simulink model "Planner_Operational_Space"  (Simulink 9.3)
settings: Solver=FixedStepDiscrete  StartTime=0.0  StopTime=stop_time  FixedStep=dt  RelTol=1e-3  EnableMultiTasking=on
values from neighbouring files (symbols this model uses):
  Cost = [0.25 0.2 0.25 0.3 start_time1 stop_time1 ]    [initialization.m]
  Cost1 = [0.25 0.3 0.25 0.25 start_time2 stop_time2 ]    [initialization.m]
  Cost2 = [0.25 0.25 0.25 0.2 start_time3 stop_time3 ]    [initialization.m]
  stop_time1 = 4    [initialization.m]
  stop_time2 = 8    [initialization.m]
undefined symbols (not defined in the file or in its folder): circonferenza1, circonferenza2, percorso
libraries: simulink x1
settings Model: Creator=Nino  LastModifiedBy=Simone
settings DataIOCC: LimitDataPoints=on
settings OptimizationCC: ExpressionDepthLimit=2147483647  InitFltsAndDblsToZero=on
settings DebuggingCC: SolverPrmCheckMsg=warning  StateNameClashWarn=warning  PregeneratedLibrarySubsystemCodeDiagnostic=none
settings GRTTargetCC: GeneratePreprocessorConditionals=Disable all
settings ConfigComp: CovSFcnEnable=off

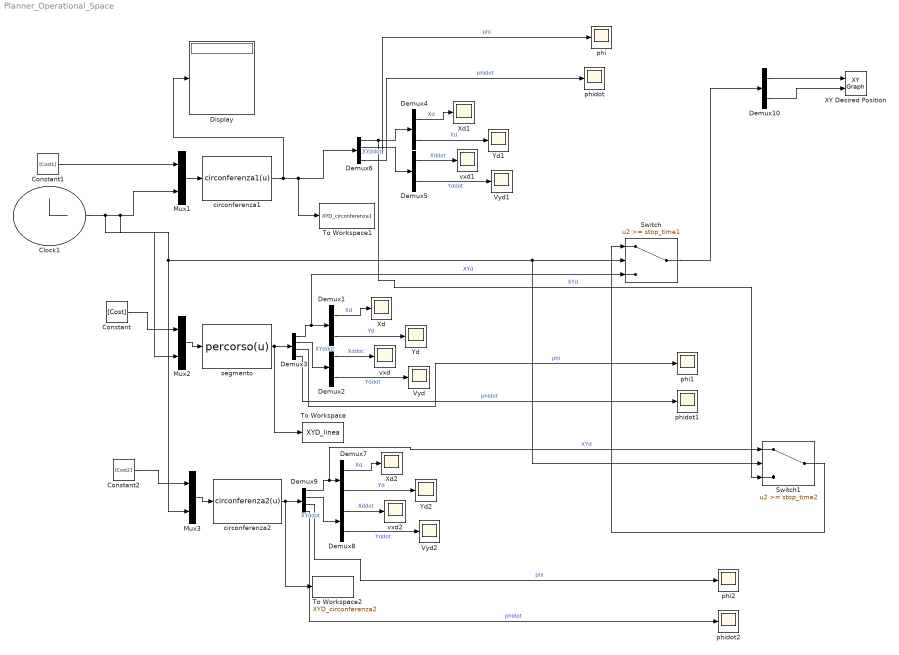
== system Planner_Operational_Space ==
  Clock1 : Clock
  Constant : Constant  Value=[Cost]
  Constant1 : Constant  Value=[Cost1]
  Constant2 : Constant  Value=[Cost2]
  Demux{1..2,4..5,7..8,10} (7 alike) : Demux  Outputs=2
  Demux3 : Demux
  Demux6 : Demux
  Demux9 : Demux
  Display : Display
  Mux1 : Mux  Inputs=2
  Mux2 : Mux  Inputs=2
  Mux3 : Mux  Inputs=2
  Switch : Switch  Threshold=stop_time1
  Switch1 : Switch  Threshold=stop_time2
  To Workspace : ToWorkspace  VariableName=XYD_linea  SaveFormat=Structure  SampleTime=-1
  To Workspace1 : ToWorkspace  VariableName=XYD_circonferenza1  SaveFormat=Structure  SampleTime=-1
  To Workspace2 : ToWorkspace  VariableName=XYD_circonferenza2  SaveFormat=Structure  SampleTime=-1
  Vyd : Scope
  Vyd1 : Scope
  Vyd2 : Scope
  "XY Desired Position " : simulink/Sinks/XY Graph  xmin=0  xmax=0.3  ymin=0  ymax=0.3  st=-1
  Xd : Scope
  Xd1 : Scope
  Xd2 : Scope
  Yd : Scope
  Yd1 : Scope
  Yd2 : Scope
  "circonferenza1  " : MATLABFcn  MATLABFcn=circonferenza1(u)  OutputDimensions=6
  circonferenza2 : MATLABFcn  MATLABFcn=circonferenza2(u)  OutputDimensions=6
  phi : Scope
  phi1 : Scope
  phi2 : Scope
  phidot : Scope
  phidot1 : Scope
  phidot2 : Scope
  segmento : MATLABFcn  MATLABFcn=percorso(u)  OutputDimensions=6
  vxd : Scope
  vxd1 : Scope
  vxd2 : Scope
  wires:
  Demux2/2 -> Vyd/1  "Yddot"
  Demux2/1 -> vxd/1  "Xddot"
  Demux1/2 -> Yd/1  "Yd"
  Demux1/1 -> Xd/1  "Xd"
  Demux3/1 -> Switch/3, Demux1/1  "XYd"
  Demux3/2 -> Demux2/1  "XYddot"
  segmento/1 -> Demux3/1, To Workspace/1
  Mux2/1 -> segmento/1
  Constant/1 -> Mux2/1
  Constant1/1 -> Mux1/1
  Mux1/1 -> "circonferenza1  "/1
  Demux4/2 -> Yd1/1  "Yd"
  "circonferenza1  "/1 -> Display/1, To Workspace1/1, Demux6/1
  Demux6/2 -> Demux5/1  "XYddot"
  Demux4/1 -> Xd1/1  "Xd"
  Demux5/2 -> Vyd1/1  "Yddot"
  Demux6/1 -> Switch1/3, Demux4/1  "XYd"
  Demux5/1 -> vxd1/1  "Xddot"
  Demux7/2 -> Yd2/1  "Yd"
  Constant2/1 -> Mux3/1
  circonferenza2/1 -> Demux9/1, To Workspace2/1
  Demux9/2 -> Demux8/1  "XYddot"
  Demux8/2 -> Vyd2/1  "Yddot"
  Demux7/1 -> Xd2/1  "Xd"
  Mux3/1 -> circonferenza2/1
  Demux9/1 -> Switch1/1, Demux7/1  "XYd"
  Demux8/1 -> vxd2/1  "Xddot"
  Demux6/3 -> phi/1  "phi"
  Demux6/4 -> phidot/1  "phidot"
  Demux3/4 -> phidot1/1  "phidot"
  Demux3/3 -> phi1/1  "phi"
  Demux9/4 -> phidot2/1  "phidot"
  Demux9/3 -> phi2/1  "phi"
  Clock1/1 -> Mux3/2, Switch1/2, Switch/2, Mux1/2, Mux2/2
  Switch/1 -> Demux10/1
  Demux10/1 -> "XY Desired Position "/1
  Demux10/2 -> "XY Desired Position "/2
  Switch1/1 -> Switch/1
